simulink model "ControlHW3"  (R2018a)
settings: Solver=VariableStepAuto  StartTime=0.0  StopTime=10.0  RelTol=1e-3
undefined symbols (not defined in the file): k_alpha, k_d, k_delta, k_phi, k_w, L, servo_Rigging_Angle, v_max
libraries: dspfdesign x3
settings Model: Creator=tagedas  LastModifiedBy=tagedas

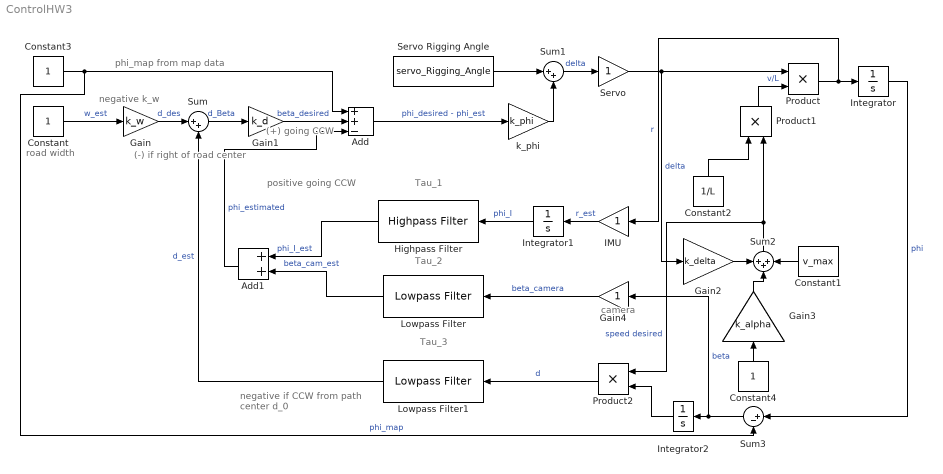
== system ControlHW3 ==
  note: camera
  note: (+) going CCW
  note: positive going CCW
  note: (-) if right of road center
  note: negative if CCW from path center d_0
  note: road width
  note: Tau_3
  note: Tau_2
  note: Tau_1
  note: negative k_w
  note: phi_map from map data
  Add : Sum  Inputs=++-
  Add1 : Sum
  Constant : Constant
  Constant1 : Constant  Value=v_max
  Constant2 : Constant  Value=1/L
  Constant3 : Constant
  Constant4 : Constant
  Gain : Gain  Gain=k_w
  Gain1 : Gain  Gain=k_d
  Gain2 : Gain  Gain=k_delta
  Gain3 : Gain  Gain=k_alpha
  Gain4 : Gain
  Highpass Filter : dspfdesign/Highpass Filter  FilterType=FIR  DesignForMinimumOrder=on  FilterOrder=50  StopbandFrequency=8e3  PassbandFrequency=12e3  StopbandAttenuation=80  PassbandRipple=0.1  InheritSampleRate=off  SampleRate=44100  SimulateUsing=Interpreted execution  roundingMode=Floor  coeffsDataTypeStr=fixdt(1,16)
      settings: SourceProductName=DSP System Toolbox
  IMU : Gain
  Integrator : Integrator
  Integrator1 : Integrator
  Integrator2 : Integrator
  Lowpass Filter : dspfdesign/Lowpass Filter  FilterType=FIR  DesignForMinimumOrder=on  FilterOrder=50  PassbandFrequency=8e3  StopbandFrequency=12e3  PassbandRipple=0.1  StopbandAttenuation=80  InheritSampleRate=off  SampleRate=44100  SimulateUsing=Interpreted execution  roundingMode=Floor  coeffsDataTypeStr=fixdt(1,16)
  Lowpass Filter1 : dspfdesign/Lowpass Filter  FilterType=FIR  DesignForMinimumOrder=on  FilterOrder=50  PassbandFrequency=8e3  StopbandFrequency=12e3  PassbandRipple=0.1  StopbandAttenuation=80  InheritSampleRate=off  SampleRate=44100  SimulateUsing=Interpreted execution  roundingMode=Floor  coeffsDataTypeStr=fixdt(1,16)
  Product : Product
  Product1 : Product
  Product2 : Product
  Servo : Gain
  Servo Rigging Angle : Constant  Value=servo_Rigging_Angle
  Sum : Sum  Inputs=|++
  Sum1 : Sum  Inputs=|++
  Sum2 : Sum  Inputs=+++
  Sum3 : Sum  Inputs=|+-
  k_phi : Gain  Gain=k_phi
  wires:
  Gain/1 -> Sum/1  "d_des"
  Sum/1 -> Gain1/1  "d_Beta"
  Lowpass Filter1/1 -> Sum/2  "d_est"
  Gain1/1 -> Add/2  "beta_desired"
  Constant/1 -> Gain/1  "w_est"
  Add/1 -> k_phi/1  "phi_desired - phi_est"
  k_phi/1 -> Sum1/2
  Servo Rigging Angle/1 -> Sum1/1
  Sum1/1 -> Servo/1  "delta"
  Servo/1 -> Product/1, Gain2/1  "delta"
  Product1/1 -> Product/2  "v/L"
  Constant2/1 -> Product1/1
  Gain2/1 -> Sum2/1
  Constant1/1 -> Sum2/3
  Sum2/1 -> Product2/1, Product1/2  "speed desired"
  Gain3/1 -> Sum2/2
  Product/1 -> IMU/1, Integrator/1  "r"
  IMU/1 -> Integrator1/1  "r_est"
  Integrator1/1 -> Highpass Filter/1  "phi_I"
  Highpass Filter/1 -> Add1/1  "phi_I_est"
  Lowpass Filter/1 -> Add1/2  "beta_cam_est"
  Add1/1 -> Add/3  "phi_estimated"
  Integrator/1 -> Sum3/1  "phi"
  Constant4/1 -> Gain3/1
  Gain4/1 -> Lowpass Filter/1  "beta_camera"
  Sum3/1 -> Integrator2/1, Gain4/1  "beta"
  Integrator2/1 -> Product2/2
  Product2/1 -> Lowpass Filter1/1  "d"
  Constant3/1 -> Sum3/2, Add/1  "phi_map"
